simulink model "rect_model"  (R2024b)
settings: Solver=VariableStepAuto  StartTime=0.0  StopTime=25.0  RelTol=1e-3
values from neighbouring files (symbols this model uses):
  A_rect = [0 0 ... (first row only)    [rect_test.m]
  B_rect = [(1/1685) -1.23 ... (first row only)    [rect_test.m]
settings Model: Creator=ananth  LastModifiedBy=ananth

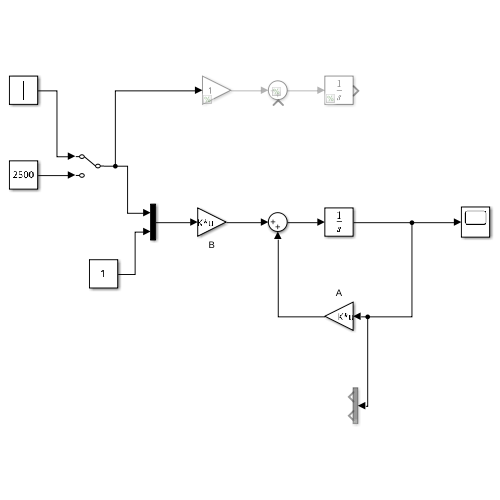
[thumbnail: Simulink's stored preview of the top-level diagram]
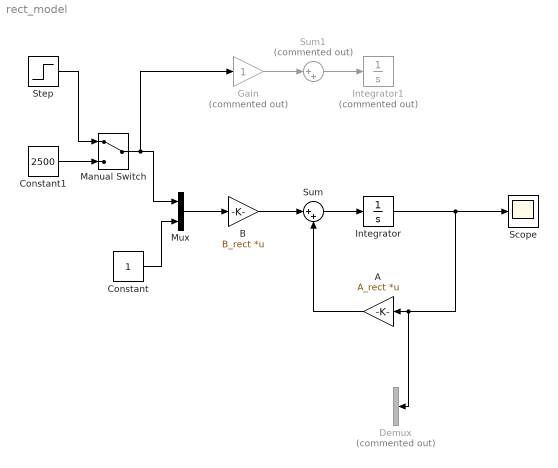
== system rect_model ==
  A : Gain  Gain=A_rect  Multiplication=Matrix(K*u)
  B : Gain  Gain=B_rect  Multiplication=Matrix(K*u)
  Constant : Constant
  Constant1 : Constant  Value=2500
  Demux : Demux  Commented=on  Outputs=2
  Gain : Gain  Commented=on
  Integrator : Integrator
  Integrator1 : Integrator  Commented=on
  Manual Switch : ManualSwitch
  Mux : Mux  Inputs=2
  Scope : Scope
  Step : Step  Time=5.0  After=3000  SampleTime=0
  Sum : Sum  Inputs=|++
  Sum1 : Sum  Commented=on  Inputs=|++
  wires:
  A/1 -> Sum/2
  B/1 -> Sum/1
  Sum/1 -> Integrator/1
  Mux/1 -> B/1
  Constant/1 -> Mux/2
  Integrator/1 -> Scope/1, Demux/1, A/1
  Constant1/1 -> Manual Switch/2
  Manual Switch/1 -> Gain/1, Mux/1
  Step/1 -> Manual Switch/1
  Gain/1 -> Sum1/1
  Sum1/1 -> Integrator1/1
